simulink model "softMBD_old"  (R2025b)
settings: Solver=FixedStepAuto  StartTime=0.0  StopTime=10  FixedStep=0.005  RelTol=1e-3
values from neighbouring files (symbols this model uses):
  FPV_mass = 0.8    [Soft.m]
  g = 9.81    [Soft.m]
  ks = 0    [Soft.m]
  p_0 = 1013.25    [Soft.m]
  Q2Ts = forcetomotors()    [Soft.m]    (also in forcetomotors.m = inv(Ts2Q))
  takeOffDuration = 2    [Soft.m]
  Ts = 0.005    [Soft.m]
undefined symbols (not defined in the file or in its folder): DiscIntNeverNeededParam, kd_pq, kd_pr, kd_y, ki_pq, ki_pr, ki_t, ki_y, kp_pq, kp_pr, kp_y, pInitialization
libraries: simulink x35, discretizing x11, slpidlib x2, shared6dof x1, dynamicsLibrary x1, aerolibasang x1, aerolibnav x1
(part 18 of 20)

== system softMBD_old/FCS/filters/Subsystem1/roll_kalman/Kalman Filter/CalculatePL ==
  A : Inport
  C : Inport  Port=2
  Qbar : Inport  Port=3
  Rbar : Inport  Port=4
  Nbar : Inport  Port=5
  Enable : Inport  Port=6
  P[k-1] : Inport  Port=7
  CovarianceZ : Constant  Value=pInitialization.Z
  DataTypeConversionL : Subsystem  AncestorBlock=|  mask(Conversion Inherited){ConvertRealWorld=Real World Value, RndMeth=Floor, DoSatur=off}
      | simulink/Signal
      | Attributes/Data Type
      | Conversion
      | Inherited
      mask prompts: ConvertRealWorld "Simulink:masks:InputAndOutputToHaveEqual_MP"; RndMeth "Simulink:masks:IntegerRoundingMode_MP"; DoSatur "Simulink:masks:SaturateToMaxOrMinWhenOverflowsOccur_MP"
      mask help: Simulink:masks:ConversionInherited_MD
      mask init: same as softMBD_old/FCS/filters/Subsystem1/pitch_kalman/Kalman Filter1/DataTypeConversionP
      mask TypeOptions ConvertRealWorld: Simulink:masks:RealWorldValue | Simulink:masks:StoredInteger
      mask TypeOptions RndMeth: Simulink:masks:Ceiling | Simulink:masks:Convergent | Simulink:masks:Floor | Simulink:masks:Nearest | Simulink:masks:Round | Simulink:masks:Simplest | Simulink:masks:Zero
      mask Display:
      | port_label('Input',2,'u');
      | port_label('Output',1,'y');
      |     if(get_param(gcbh,'ConvertRealWorld') == "Stored Integer")
      |        disp('SI')
      |     else
      |        disp('Convert')
      |     end
  DataTypeConversionM : Subsystem  AncestorBlock=|  mask(Conversion Inherited){ConvertRealWorld=Real World Value, RndMeth=Floor, DoSatur=off}
      | simulink/Signal
      | Attributes/Data Type
      | Conversion
      | Inherited
      mask prompts: ConvertRealWorld "Simulink:masks:InputAndOutputToHaveEqual_MP"; RndMeth "Simulink:masks:IntegerRoundingMode_MP"; DoSatur "Simulink:masks:SaturateToMaxOrMinWhenOverflowsOccur_MP"
      mask help: Simulink:masks:ConversionInherited_MD
      mask init: same as softMBD_old/FCS/filters/Subsystem1/pitch_kalman/Kalman Filter1/DataTypeConversionP
      mask TypeOptions ConvertRealWorld: Simulink:masks:RealWorldValue | Simulink:masks:StoredInteger
      mask TypeOptions RndMeth: Simulink:masks:Ceiling | Simulink:masks:Convergent | Simulink:masks:Floor | Simulink:masks:Nearest | Simulink:masks:Round | Simulink:masks:Simplest | Simulink:masks:Zero
      mask Display:
      | port_label('Input',2,'u');
      | port_label('Output',1,'y');
      |     if(get_param(gcbh,'ConvertRealWorld') == "Stored Integer")
      |        disp('SI')
      |     else
      |        disp('Convert')
      |     end
  DataTypeConversionP : Subsystem  AncestorBlock=|  mask(Conversion Inherited){ConvertRealWorld=Real World Value, RndMeth=Floor, DoSatur=off}
      | simulink/Signal
      | Attributes/Data Type
      | Conversion
      | Inherited
      mask prompts: ConvertRealWorld "Simulink:masks:InputAndOutputToHaveEqual_MP"; RndMeth "Simulink:masks:IntegerRoundingMode_MP"; DoSatur "Simulink:masks:SaturateToMaxOrMinWhenOverflowsOccur_MP"
      mask help: Simulink:masks:ConversionInherited_MD
      mask init: same as softMBD_old/FCS/filters/Subsystem1/pitch_kalman/Kalman Filter1/DataTypeConversionP
      mask TypeOptions ConvertRealWorld: Simulink:masks:RealWorldValue | Simulink:masks:StoredInteger
      mask TypeOptions RndMeth: Simulink:masks:Ceiling | Simulink:masks:Convergent | Simulink:masks:Floor | Simulink:masks:Nearest | Simulink:masks:Round | Simulink:masks:Simplest | Simulink:masks:Zero
      mask Display:
      | port_label('Input',2,'u');
      | port_label('Output',1,'y');
      |     if(get_param(gcbh,'ConvertRealWorld') == "Stored Integer")
      |        disp('SI')
      |     else
      |        disp('Convert')
      |     end
  DataTypeConversionZ : Subsystem  AncestorBlock=|  mask(Conversion Inherited){ConvertRealWorld=Real World Value, RndMeth=Floor, DoSatur=off}
      | simulink/Signal
      | Attributes/Data Type
      | Conversion
      | Inherited
      mask prompts: ConvertRealWorld "Simulink:masks:InputAndOutputToHaveEqual_MP"; RndMeth "Simulink:masks:IntegerRoundingMode_MP"; DoSatur "Simulink:masks:SaturateToMaxOrMinWhenOverflowsOccur_MP"
      mask help: Simulink:masks:ConversionInherited_MD
      mask init: same as softMBD_old/FCS/filters/Subsystem1/pitch_kalman/Kalman Filter1/DataTypeConversionP
      mask TypeOptions ConvertRealWorld: Simulink:masks:RealWorldValue | Simulink:masks:StoredInteger
      mask TypeOptions RndMeth: Simulink:masks:Ceiling | Simulink:masks:Convergent | Simulink:masks:Floor | Simulink:masks:Nearest | Simulink:masks:Round | Simulink:masks:Simplest | Simulink:masks:Zero
      mask Display:
      | port_label('Input',2,'u');
      | port_label('Output',1,'y');
      |     if(get_param(gcbh,'ConvertRealWorld') == "Stored Integer")
      |        disp('SI')
      |     else
      |        disp('Convert')
      |     end
  Ground : Subsystem  AncestorBlock=ctrlSharedLib/Utilities/Ground  mask(ctrlSharedLibGround){OutDataTypeStr=single, Dimensions=1}
      mask prompts: OutDataTypeStr "Simulink:blkprm_prompts:UNIFIEDDATATYPE"; Dimensions "Simulink:blkprm_prompts:SigSpecDims"
      mask TypeOptions OutDataTypeStr: Signal Specification/OutDataTypeStr
      mask TypeOptions Dimensions: Signal Specification/Dimensions
      mask DialogControl OutDataTypeStr Prompt: Data type:
      mask DialogControl Dimensions Prompt: Dimensions (-1 for inherited):
  KalmanGainL : Constant  Value=pInitialization.L
  KalmanGainM : Constant  Value=pInitialization.M
  Terminator{,2,4..8} (7 alike) : Terminator
  M : Outport  VectorParamsAs1DForOutWhenUnconnected=off
  L : Outport  Port=2  VectorParamsAs1DForOutWhenUnconnected=off
  Z : Outport  Port=3  VectorParamsAs1DForOutWhenUnconnected=off
  P : Outport  Port=4  VectorParamsAs1DForOutWhenUnconnected=off
  wires:
  DataTypeConversionP/1(y) -> P/1
  CovarianceZ/1 -> DataTypeConversionZ/2(u)
  DataTypeConversionZ/1(y) -> Z/1
  Ground/1(Out) -> DataTypeConversionP/2(u)
  DataTypeConversionM/1(y) -> M/1
  KalmanGainM/1 -> DataTypeConversionM/2(u)
  P[k-1]/1 -> Terminator8/1
  Enable/1 -> Terminator7/1
  KalmanGainL/1 -> DataTypeConversionL/2(u)
  DataTypeConversionL/1(y) -> L/1
  Nbar/1 -> Terminator6/1
  Rbar/1 -> Terminator5/1
  Qbar/1 -> Terminator4/1
  C/1 -> Terminator2/1, DataTypeConversionL/1(DTS reference), DataTypeConversionM/1(DTS reference), DataTypeConversionZ/1(DTS reference), DataTypeConversionP/1(DTS reference)
  A/1 -> Terminator/1

== system softMBD_old/FCS/filters/Subsystem1/roll_kalman/Kalman Filter/CalculateYhat ==
  u : Inport  SampleTime=pInitialization.Ts
  C : Inport  Port=2  SampleTime=pInitialization.Ts
  D : Inport  Port=3  SampleTime=pInitialization.Ts
  xhat : Inport  Port=4  SampleTime=pInitialization.Ts
  Ground : Subsystem  AncestorBlock=ctrlSharedLib/Utilities/Ground  mask(ctrlSharedLibGround){OutDataTypeStr=single, Dimensions=1}
      mask prompts: OutDataTypeStr "Simulink:blkprm_prompts:UNIFIEDDATATYPE"; Dimensions "Simulink:blkprm_prompts:SigSpecDims"
      mask TypeOptions OutDataTypeStr: Signal Specification/OutDataTypeStr
      mask TypeOptions Dimensions: Signal Specification/Dimensions
      mask DialogControl OutDataTypeStr Prompt: Data type:
      mask DialogControl Dimensions Prompt: Dimensions (-1 for inherited):
  TerminatorC : Terminator
  TerminatorD : Terminator
  Terminatoru : Terminator
  Terminatorxhat : Terminator
  y[.] : Outport  VectorParamsAs1DForOutWhenUnconnected=off
  wires:
  Ground/1(Out) -> y[.]/1
  u/1 -> Terminatoru/1
  D/1 -> TerminatorD/1
  xhat/1 -> Terminatorxhat/1
  C/1 -> TerminatorC/1

== system softMBD_old/FCS/filters/Subsystem1/roll_kalman/Kalman Filter/CovarianceOutputConfigurator ==
  Z : Inport
  P : Inport  Port=2
  TerminatorP : Terminator
  TerminatorZ : Terminator
  decideOutput : Subsystem  mask(outputZorP){}
  Covariance : Outport  VectorParamsAs1DForOutWhenUnconnected=off
  wires:
  decideOutput/1(P) -> Covariance/1
  P/1 -> TerminatorP/1
  Z/1 -> TerminatorZ/1, decideOutput/1(Z)

== system softMBD_old/FCS/filters/Subsystem1/roll_kalman/Kalman Filter/DataTypeConversionA ==
  typeRef : Inport
  u : Inport  Port=2
  Data Type Duplicate : DataTypeDuplicate
  u_ : Outport  VectorParamsAs1DForOutWhenUnconnected=off
  wires:
  typeRef/1 -> Data Type Duplicate/1
  u/1 -> Data Type Duplicate/2, u_/1

== system softMBD_old/FCS/filters/Subsystem1/roll_kalman/Kalman Filter/DataTypeConversionB ==
  typeRef : Inport
  u : Inport  Port=2
  Data Type Duplicate : DataTypeDuplicate
  u_ : Outport  VectorParamsAs1DForOutWhenUnconnected=off
  wires:
  typeRef/1 -> Data Type Duplicate/1
  u/1 -> Data Type Duplicate/2, u_/1

== system softMBD_old/FCS/filters/Subsystem1/roll_kalman/Kalman Filter/DataTypeConversionC ==
  typeRef : Inport
  u : Inport  Port=2
  Data Type Duplicate : DataTypeDuplicate
  u_ : Outport  VectorParamsAs1DForOutWhenUnconnected=off
  wires:
  typeRef/1 -> Data Type Duplicate/1
  u/1 -> Data Type Duplicate/2, u_/1

== system softMBD_old/FCS/filters/Subsystem1/roll_kalman/Kalman Filter/DataTypeConversionD ==
  typeRef : Inport
  u : Inport  Port=2
  Data Type Duplicate : DataTypeDuplicate
  u_ : Outport  VectorParamsAs1DForOutWhenUnconnected=off
  wires:
  typeRef/1 -> Data Type Duplicate/1
  u/1 -> Data Type Duplicate/2, u_/1

== system softMBD_old/FCS/filters/Subsystem1/roll_kalman/Kalman Filter/DataTypeConversionEnable ==
  u : Inport
  u_ : Outport  VectorParamsAs1DForOutWhenUnconnected=off
  wires:
  u/1 -> u_/1

== system softMBD_old/FCS/filters/Subsystem1/roll_kalman/Kalman Filter/DataTypeConversionG ==
  typeRef : Inport
  u : Inport  Port=2
  Data Type Duplicate : DataTypeDuplicate
  u_ : Outport  VectorParamsAs1DForOutWhenUnconnected=off
  wires:
  typeRef/1 -> Data Type Duplicate/1
  u/1 -> Data Type Duplicate/2, u_/1

== system softMBD_old/FCS/filters/Subsystem1/roll_kalman/Kalman Filter/DataTypeConversionH ==
  typeRef : Inport
  u : Inport  Port=2
  Data Type Duplicate : DataTypeDuplicate
  u_ : Outport  VectorParamsAs1DForOutWhenUnconnected=off
  wires:
  typeRef/1 -> Data Type Duplicate/1
  u/1 -> Data Type Duplicate/2, u_/1

== system softMBD_old/FCS/filters/Subsystem1/roll_kalman/Kalman Filter/DataTypeConversionN ==
  typeRef : Inport
  u : Inport  Port=2
  Data Type Duplicate : DataTypeDuplicate
  u_ : Outport  VectorParamsAs1DForOutWhenUnconnected=off
  wires:
  typeRef/1 -> Data Type Duplicate/1
  u/1 -> Data Type Duplicate/2, u_/1

== system softMBD_old/FCS/filters/Subsystem1/roll_kalman/Kalman Filter/DataTypeConversionP ==
  DTS reference : Inport
  u : Inport  Port=2
  Conversion : DataTypeConversion  SaturateOnIntegerOverflow=off  RndMeth=Floor  LockScale=on
  Data Type Duplicate : DataTypeDuplicate  DisableCoverage=on
  y : Outport
  wires:
  Conversion/1 -> Data Type Duplicate/2, y/1
  DTS reference/1 -> Data Type Duplicate/1
  u/1 -> Conversion/1

== system softMBD_old/FCS/filters/Subsystem1/roll_kalman/Kalman Filter/DataTypeConversionP0 ==
  typeRef : Inport
  u : Inport  Port=2
  Data Type Duplicate : DataTypeDuplicate
  u_ : Outport  VectorParamsAs1DForOutWhenUnconnected=off
  wires:
  typeRef/1 -> Data Type Duplicate/1
  u/1 -> Data Type Duplicate/2, u_/1

== system softMBD_old/FCS/filters/Subsystem1/roll_kalman/Kalman Filter/DataTypeConversionQ ==
  typeRef : Inport
  u : Inport  Port=2
  Data Type Duplicate : DataTypeDuplicate
  u_ : Outport  VectorParamsAs1DForOutWhenUnconnected=off
  wires:
  typeRef/1 -> Data Type Duplicate/1
  u/1 -> Data Type Duplicate/2, u_/1

== system softMBD_old/FCS/filters/Subsystem1/roll_kalman/Kalman Filter/DataTypeConversionR ==
  typeRef : Inport
  u : Inport  Port=2
  Data Type Duplicate : DataTypeDuplicate
  u_ : Outport  VectorParamsAs1DForOutWhenUnconnected=off
  wires:
  typeRef/1 -> Data Type Duplicate/1
  u/1 -> Data Type Duplicate/2, u_/1

== system softMBD_old/FCS/filters/Subsystem1/roll_kalman/Kalman Filter/DataTypeConversionReset ==
  u : Inport
  u_ : Outport  VectorParamsAs1DForOutWhenUnconnected=off
  wires:
  u/1 -> u_/1

== system softMBD_old/FCS/filters/Subsystem1/roll_kalman/Kalman Filter/DataTypeConversionX ==
  DTS reference : Inport
  u : Inport  Port=2
  Conversion : DataTypeConversion  SaturateOnIntegerOverflow=off  RndMeth=Floor  LockScale=on
  Data Type Duplicate : DataTypeDuplicate  DisableCoverage=on
  y : Outport
  wires:
  Conversion/1 -> Data Type Duplicate/2, y/1
  DTS reference/1 -> Data Type Duplicate/1
  u/1 -> Conversion/1

== system softMBD_old/FCS/filters/Subsystem1/roll_kalman/Kalman Filter/DataTypeConversionX0 ==
  typeRef : Inport
  u : Inport  Port=2
  Data Type Duplicate : DataTypeDuplicate
  u_ : Outport  VectorParamsAs1DForOutWhenUnconnected=off
  wires:
  typeRef/1 -> Data Type Duplicate/1
  u/1 -> Data Type Duplicate/2, u_/1

== system softMBD_old/FCS/filters/Subsystem1/roll_kalman/Kalman Filter/DataTypeConversionu ==
  In1 : Inport
  u : Inport  Port=2
  Terminator : Terminator
  u_ : Outport  VectorParamsAs1DForOutWhenUnconnected=off
  wires:
  In1/1 -> Terminator/1
  u/1 -> u_/1

== system softMBD_old/FCS/filters/Subsystem1/roll_kalman/Kalman Filter/MemoryP ==
  T : Inport
  P : Inport  Port=2
  Terminator : Terminator
  P_ : Outport  VectorParamsAs1DForOutWhenUnconnected=off
  wires:
  T/1 -> Terminator/1
  P/1 -> P_/1

== system softMBD_old/FCS/filters/Subsystem1/roll_kalman/Kalman Filter/Observer ==
  note: A*xhat+B*u+L*(yMeas-yHat)
      | or
      | A*xhat+B*u
  u[k] : Inport  SampleTime=pInitialization.Ts
  y[k] : Inport  Port=2  SampleTime=pInitialization.Ts
  A[k] : Inport  Port=3  SampleTime=pInitialization.Ts
  B[k] : Inport  Port=4  SampleTime=pInitialization.Ts
  C[k] : Inport  Port=5  SampleTime=pInitialization.Ts
  D[k] : Inport  Port=6  SampleTime=pInitialization.Ts
  L[k] : Inport  Port=7  SampleTime=pInitialization.Ts
  Enable : Inport  Port=8  SampleTime=pInitialization.Ts
  xhat[k|k-1] : Inport  Port=9  SampleTime=pInitialization.Ts
  A[k]*xhat[k|k-1] : Product  Multiplication=Matrix(*)
  Add : Sum  Inputs=+++
  B[k]*u[k] : Product  Multiplication=Matrix(*)
  MeasurementUpdate : Subsystem  TreatAsAtomicUnit=on
  Reshape : Reshape
  x[k+1|k] : Outport  SampleTime=pInitialization.Ts  VectorParamsAs1DForOutWhenUnconnected=off
  wires:
  D[k]/1 -> MeasurementUpdate/5(D[k])
  Reshape/1 -> x[k+1|k]/1
  y[k]/1 -> MeasurementUpdate/2(y[k])
  C[k]/1 -> MeasurementUpdate/3(C[k])
  MeasurementUpdate/1(L*(y[k]-yhat[k|k-1])) -> Add/3
  A[k]/1 -> A[k]*xhat[k|k-1]/1
  xhat[k|k-1]/1 -> A[k]*xhat[k|k-1]/2, MeasurementUpdate/4(xhat[k|k-1])
  B[k]/1 -> B[k]*u[k]/1
  L[k]/1 -> MeasurementUpdate/1(L[k])
  A[k]*xhat[k|k-1]/1 -> Add/2
  u[k]/1 -> B[k]*u[k]/2, MeasurementUpdate/6(u[k])
  Add/1 -> Reshape/1
  B[k]*u[k]/1 -> Add/1
  Enable/1 -> MeasurementUpdate/Enable

== system softMBD_old/FCS/filters/Subsystem1/roll_kalman/Kalman Filter/ReducedQRN ==
  G : Inport  SampleTime=pInitialization.Ts
  H : Inport  Port=2  SampleTime=pInitialization.Ts
  Q : Inport  Port=3  SampleTime=pInitialization.Ts
  R : Inport  Port=4  SampleTime=pInitialization.Ts
  N : Inport  Port=5  SampleTime=pInitialization.Ts
  Ground : Subsystem  AncestorBlock=ctrlSharedLib/Utilities/Ground  mask(ctrlSharedLibGround){OutDataTypeStr=single, Dimensions=1}
      mask prompts: OutDataTypeStr "Simulink:blkprm_prompts:UNIFIEDDATATYPE"; Dimensions "Simulink:blkprm_prompts:SigSpecDims"
      mask TypeOptions OutDataTypeStr: Signal Specification/OutDataTypeStr
      mask TypeOptions Dimensions: Signal Specification/Dimensions
      mask DialogControl OutDataTypeStr Prompt: Data type:
      mask DialogControl Dimensions Prompt: Dimensions (-1 for inherited):
  Terminator{,1..4} (5 alike) : Terminator
  Qbar : Outport  SampleTime=pInitialization.Ts  VectorParamsAs1DForOutWhenUnconnected=off
  Rbar : Outport  Port=2  SampleTime=pInitialization.Ts  VectorParamsAs1DForOutWhenUnconnected=off
  Nbar : Outport  Port=3  SampleTime=pInitialization.Ts  VectorParamsAs1DForOutWhenUnconnected=off
  wires:
  Ground/1(Out) -> Rbar/1, Nbar/1, Qbar/1
  N/1 -> Terminator4/1
  R/1 -> Terminator3/1
  Q/1 -> Terminator2/1
  H/1 -> Terminator1/1
  G/1 -> Terminator/1

== system softMBD_old/FCS/filters/Subsystem1/roll_kalman/Kalman Filter/Reset ==
  note: Specification is to avoid underspecified data type warnings in the code generation process
  Ground : Ground
  Signal Specification : SignalSpecification  OutDataTypeStr=boolean  Dimensions=1
  Out : Outport  VectorParamsAs1DForOutWhenUnconnected=off
  wires:
  Signal Specification/1 -> Out/1
  Ground/1 -> Signal Specification/1

== system softMBD_old/FCS/filters/Subsystem1/roll_kalman/Kalman Filter/Reshapeyhat ==
  u : Inport
  u_ : Outport  VectorParamsAs1DForOutWhenUnconnected=off
  wires:
  u/1 -> u_/1

== system softMBD_old/FCS/filters/Subsystem1/roll_kalman/Kalman Filter/ScalarExpansionP0 ==
  u : Inport
  u_ : Outport  VectorParamsAs1DForOutWhenUnconnected=off
  wires:
  u/1 -> u_/1

== system softMBD_old/FCS/filters/Subsystem1/roll_kalman/Kalman Filter/ScalarExpansionQ ==
  u : Inport
  u_ : Outport  VectorParamsAs1DForOutWhenUnconnected=off
  wires:
  u/1 -> u_/1

== system softMBD_old/FCS/filters/Subsystem1/roll_kalman/Kalman Filter/ScalarExpansionR ==
  u : Inport
  u_ : Outport  VectorParamsAs1DForOutWhenUnconnected=off
  wires:
  u/1 -> u_/1

== system softMBD_old/FCS/filters/Subsystem1/roll_kalman/Kalman Filter/UseCurrentEstimator ==
  note: System model has D=0
      | Break connection, avoid fictitious algebraic loop
  Enable[k] : Inport  SampleTime=pInitialization.Ts
  M[k] : Inport  Port=2  SampleTime=pInitialization.Ts
  u (unused) : Inport  Port=3  SampleTime=pInitialization.Ts
  y[k] : Inport  Port=4  SampleTime=pInitialization.Ts
  C[k] : Inport  Port=5  SampleTime=pInitialization.Ts
  D (unused) : Inport  Port=6  SampleTime=pInitialization.Ts
  xhat[k|k-1] : Inport  Port=7  SampleTime=pInitialization.Ts
  Add : Sum
  Enabled Subsystem : Subsystem  TreatAsAtomicUnit=on
  Terminator : Terminator
  Terminator1 : Terminator
  xhat[k|k] : Outport  SampleTime=pInitialization.Ts  VectorParamsAs1DForOutWhenUnconnected=off
  wires:
  Add/1 -> xhat[k|k]/1
  u (unused)/1 -> Terminator1/1
  D (unused)/1 -> Terminator/1
  M[k]/1 -> Enabled Subsystem/1(M[k])
  C[k]/1 -> Enabled Subsystem/2(C[k])
  y[k]/1 -> Enabled Subsystem/3(y[k])
  xhat[k|k-1]/1 -> Add/2, Enabled Subsystem/4(xhat[k|k-1])
  Enabled Subsystem/1(deltax) -> Add/1
  Enable[k]/1 -> Enabled Subsystem/Enable

== system softMBD_old/FCS/filters/Subsystem1/roll_kalman/Kalman Filter/checkA ==
  In1 : Inport
  u : Inport  Port=2
  Terminator : Terminator
  u_ : Outport  VectorParamsAs1DForOutWhenUnconnected=off
  wires:
  In1/1 -> Terminator/1
  u/1 -> u_/1

== system softMBD_old/FCS/filters/Subsystem1/roll_kalman/Kalman Filter/checkB ==
  In1 : Inport
  u : Inport  Port=2
  Terminator : Terminator
  u_ : Outport  VectorParamsAs1DForOutWhenUnconnected=off
  wires:
  In1/1 -> Terminator/1
  u/1 -> u_/1

== system softMBD_old/FCS/filters/Subsystem1/roll_kalman/Kalman Filter/checkC ==
  In1 : Inport
  u : Inport  Port=2
  Terminator : Terminator
  u_ : Outport  VectorParamsAs1DForOutWhenUnconnected=off
  wires:
  In1/1 -> Terminator/1
  u/1 -> u_/1

== system softMBD_old/FCS/filters/Subsystem1/roll_kalman/Kalman Filter/checkD ==
  In1 : Inport
  u : Inport  Port=2
  Terminator : Terminator
  u_ : Outport  VectorParamsAs1DForOutWhenUnconnected=off
  wires:
  In1/1 -> Terminator/1
  u/1 -> u_/1

== system softMBD_old/FCS/filters/Subsystem1/roll_kalman/Kalman Filter/checkEnable ==
  In1 : Inport
  u : Inport  Port=2
  Terminator : Terminator
  u_ : Outport  VectorParamsAs1DForOutWhenUnconnected=off
  wires:
  In1/1 -> Terminator/1
  u/1 -> u_/1

== system softMBD_old/FCS/filters/Subsystem1/roll_kalman/Kalman Filter/checkG ==
  In1 : Inport
  u : Inport  Port=2
  Terminator : Terminator
  u_ : Outport  VectorParamsAs1DForOutWhenUnconnected=off
  wires:
  In1/1 -> Terminator/1
  u/1 -> u_/1

== system softMBD_old/FCS/filters/Subsystem1/roll_kalman/Kalman Filter/checkH ==
  In1 : Inport
  u : Inport  Port=2
  Terminator : Terminator
  u_ : Outport  VectorParamsAs1DForOutWhenUnconnected=off
  wires:
  In1/1 -> Terminator/1
  u/1 -> u_/1

== system softMBD_old/FCS/filters/Subsystem1/roll_kalman/Kalman Filter/checkN ==
  In1 : Inport
  u : Inport  Port=2
  Terminator : Terminator
  u_ : Outport  VectorParamsAs1DForOutWhenUnconnected=off
  wires:
  In1/1 -> Terminator/1
  u/1 -> u_/1

== system softMBD_old/FCS/filters/Subsystem1/roll_kalman/Kalman Filter/checkP0 ==
  In1 : Inport
  u : Inport  Port=2
  Terminator : Terminator
  u_ : Outport  VectorParamsAs1DForOutWhenUnconnected=off
  wires:
  In1/1 -> Terminator/1
  u/1 -> u_/1

== system softMBD_old/FCS/filters/Subsystem1/roll_kalman/Kalman Filter/checkQ ==
  In1 : Inport
  u : Inport  Port=2
  Terminator : Terminator
  u_ : Outport  VectorParamsAs1DForOutWhenUnconnected=off
  wires:
  In1/1 -> Terminator/1
  u/1 -> u_/1

== system softMBD_old/FCS/filters/Subsystem1/roll_kalman/Kalman Filter/checkR ==
  In1 : Inport
  u : Inport  Port=2
  Terminator : Terminator
  u_ : Outport  VectorParamsAs1DForOutWhenUnconnected=off
  wires:
  In1/1 -> Terminator/1
  u/1 -> u_/1

== system softMBD_old/FCS/filters/Subsystem1/roll_kalman/Kalman Filter/checkReset ==
  In1 : Inport
  u : Inport  Port=2
  Terminator : Terminator
  u_ : Outport  VectorParamsAs1DForOutWhenUnconnected=off
  wires:
  In1/1 -> Terminator/1
  u/1 -> u_/1

== system softMBD_old/FCS/filters/Subsystem1/roll_kalman/Kalman Filter/checkX0 ==
  In1 : Inport
  u : Inport  Port=2
  Terminator : Terminator
  u_ : Outport  VectorParamsAs1DForOutWhenUnconnected=off
  wires:
  In1/1 -> Terminator/1
  u/1 -> u_/1

== system softMBD_old/FCS/filters/Subsystem1/roll_kalman/Kalman Filter/checku ==
  Ref : Inport
  u : Inport  Port=2
  CheckSignalProperties : S-Function  FunctionName=ctrlKalmanFilterCheckSignals  Parameters=parentBlockPath,portName,isContinuousTime,pInitialization.Ts,Ns,Nu,Nw,Ny  SFunctionDeploymentMode=off  EnableBusSupport=off
  Data Type Conversion3 : DataTypeConversion  OutDataTypeStr=single  SaturateOnIntegerOverflow=off  RndMeth=Floor
  y : Outport  VectorParamsAs1DForOutWhenUnconnected=off
  wires:
  u/1 -> CheckSignalProperties/2, y/1
  Ref/1 -> Data Type Conversion3/1
  Data Type Conversion3/1 -> CheckSignalProperties/1

== system softMBD_old/FCS/filters/Subsystem1/roll_kalman/Kalman Filter/checky ==
  Ref : Inport
  u : Inport  Port=2
  CheckSignalProperties : S-Function  FunctionName=ctrlKalmanFilterCheckSignals  Parameters=parentBlockPath,portName,isContinuousTime,pInitialization.Ts,Ns,Nu,Nw,Ny  SFunctionDeploymentMode=off  EnableBusSupport=off
  y : Outport  VectorParamsAs1DForOutWhenUnconnected=off
  wires:
  u/1 -> CheckSignalProperties/2, y/1
  Ref/1 -> CheckSignalProperties/1

== system softMBD_old/FCS/Controller/position_controller/PID Controller/Anti-windup/Cont. Clamping Ideal/Dead Zone ==
  preSat : Inport
  Upper Limit : Inport  Port=2  SampleTime=SampleTime
  Lower Limit : Inport  Port=3  SampleTime=SampleTime
  Disabled : Subsystem  VariantControl=Disabled
  Enabled : Subsystem  VariantControl=Enabled
  External : Subsystem  VariantControl=External
  DZ out : Outport

== system softMBD_old/FCS/Controller/position_controller/PID Controller/Anti-windup/Cont. Clamping Parallel/Dead Zone ==
  preSat : Inport
  Upper Limit : Inport  Port=2  SampleTime=SampleTime
  Lower Limit : Inport  Port=3  SampleTime=SampleTime
  Disabled : Subsystem  VariantControl=Disabled
  Enabled : Subsystem  VariantControl=Enabled
  External : Subsystem  VariantControl=External
  DZ out : Outport

== system softMBD_old/FCS/Controller/position_controller/PID Controller/Anti-windup/Disc. Clamping Ideal/Dead Zone ==
  preSat : Inport
  Upper Limit : Inport  Port=2  SampleTime=SampleTime
  Lower Limit : Inport  Port=3  SampleTime=SampleTime
  Disabled : Subsystem  VariantControl=Disabled
  Enabled : Subsystem  VariantControl=Enabled
  External : Subsystem  VariantControl=External
  DZ out : Outport

== system softMBD_old/FCS/Controller/position_controller/PID Controller/Anti-windup/Disc. Clamping Parallel/Dead Zone ==
  preSat : Inport
  Upper Limit : Inport  Port=2  SampleTime=SampleTime
  Lower Limit : Inport  Port=3  SampleTime=SampleTime
  Disabled : Subsystem  VariantControl=Disabled
  Enabled : Subsystem  VariantControl=Enabled
  External : Subsystem  VariantControl=External
  DZ out : Outport

== system softMBD_old/FCS/Controller/position_controller/PID Controller/Filter/Differentiator/Tsamp ==
  U : Inport  SampleTime=SampleTime
  Ts : Inport  Port=2  SampleTime=SampleTime
  External Ts : Subsystem  VariantControl=ExternalTs
  Internal Ts : Subsystem  VariantControl=InternalTs
  Out1 : Outport  SampleTime=SampleTime

== system softMBD_old/FCS/Controller/position_controller/PID Controller/Filter/Disc. Backward Euler Filter/Tsamp ==
  N : Inport  SampleTime=SampleTime
  Ts : Inport  Port=2  SampleTime=SampleTime
  External Ts : Subsystem  VariantControl=ExternalTs
  Internal Ts : Subsystem  VariantControl=InternalTs
  Out1 : Outport  SampleTime=SampleTime

== system softMBD_old/FCS/Controller/position_controller/PID Controller/Filter/Disc. Backward Euler Filter Only/Tsamp ==
  N : Inport  SampleTime=SampleTime
  Ts : Inport  Port=2  SampleTime=SampleTime
  External Ts : Subsystem  VariantControl=ExternalTs
  Internal Ts : Subsystem  VariantControl=InternalTs
  Out1 : Outport  SampleTime=SampleTime

== system softMBD_old/FCS/Controller/position_controller/PID Controller/Filter/Disc. Trapezoidal Filter/Tsamp ==
  N : Inport  SampleTime=SampleTime
  Ts : Inport  Port=2  SampleTime=SampleTime
  External Ts : Subsystem  VariantControl=ExternalTs
  Internal Ts : Subsystem  VariantControl=InternalTs
  Out1 : Outport  SampleTime=SampleTime

== system softMBD_old/FCS/Controller/position_controller/PID Controller/Filter/Disc. Trapezoidal Filter Only/Tsamp ==
  N : Inport  SampleTime=SampleTime
  Ts : Inport  Port=2  SampleTime=SampleTime
  External Ts : Subsystem  VariantControl=ExternalTs
  Internal Ts : Subsystem  VariantControl=InternalTs
  Out1 : Outport  SampleTime=SampleTime

== system softMBD_old/FCS/Controller/position_controller/PID Controller1/Anti-windup/Cont. Clamping Ideal/Dead Zone ==
  preSat : Inport
  Upper Limit : Inport  Port=2  SampleTime=SampleTime
  Lower Limit : Inport  Port=3  SampleTime=SampleTime
  Disabled : Subsystem  VariantControl=Disabled
  Enabled : Subsystem  VariantControl=Enabled
  External : Subsystem  VariantControl=External
  DZ out : Outport

== system softMBD_old/FCS/Controller/position_controller/PID Controller1/Anti-windup/Cont. Clamping Parallel/Dead Zone ==
  preSat : Inport
  Upper Limit : Inport  Port=2  SampleTime=SampleTime
  Lower Limit : Inport  Port=3  SampleTime=SampleTime
  Disabled : Subsystem  VariantControl=Disabled
  Enabled : Subsystem  VariantControl=Enabled
  External : Subsystem  VariantControl=External
  DZ out : Outport

== system softMBD_old/FCS/Controller/position_controller/PID Controller1/Anti-windup/Disc. Clamping Ideal/Dead Zone ==
  preSat : Inport
  Upper Limit : Inport  Port=2  SampleTime=SampleTime
  Lower Limit : Inport  Port=3  SampleTime=SampleTime
  Disabled : Subsystem  VariantControl=Disabled
  Enabled : Subsystem  VariantControl=Enabled
  External : Subsystem  VariantControl=External
  DZ out : Outport

== system softMBD_old/FCS/Controller/position_controller/PID Controller1/Anti-windup/Disc. Clamping Parallel/Dead Zone ==
  preSat : Inport
  Upper Limit : Inport  Port=2  SampleTime=SampleTime
  Lower Limit : Inport  Port=3  SampleTime=SampleTime
  Disabled : Subsystem  VariantControl=Disabled
  Enabled : Subsystem  VariantControl=Enabled
  External : Subsystem  VariantControl=External
  DZ out : Outport

== system softMBD_old/FCS/Controller/position_controller/PID Controller1/Filter/Differentiator/Tsamp ==
  U : Inport  SampleTime=SampleTime
  Ts : Inport  Port=2  SampleTime=SampleTime
  External Ts : Subsystem  VariantControl=ExternalTs
  Internal Ts : Subsystem  VariantControl=InternalTs
  Out1 : Outport  SampleTime=SampleTime

== system softMBD_old/FCS/Controller/position_controller/PID Controller1/Filter/Disc. Backward Euler Filter/Tsamp ==
  N : Inport  SampleTime=SampleTime
  Ts : Inport  Port=2  SampleTime=SampleTime
  External Ts : Subsystem  VariantControl=ExternalTs
  Internal Ts : Subsystem  VariantControl=InternalTs
  Out1 : Outport  SampleTime=SampleTime

== system softMBD_old/FCS/Controller/position_controller/PID Controller1/Filter/Disc. Backward Euler Filter Only/Tsamp ==
  N : Inport  SampleTime=SampleTime
  Ts : Inport  Port=2  SampleTime=SampleTime
  External Ts : Subsystem  VariantControl=ExternalTs
  Internal Ts : Subsystem  VariantControl=InternalTs
  Out1 : Outport  SampleTime=SampleTime

== system softMBD_old/FCS/Controller/position_controller/PID Controller1/Filter/Disc. Trapezoidal Filter/Tsamp ==
  N : Inport  SampleTime=SampleTime
  Ts : Inport  Port=2  SampleTime=SampleTime
  External Ts : Subsystem  VariantControl=ExternalTs
  Internal Ts : Subsystem  VariantControl=InternalTs
  Out1 : Outport  SampleTime=SampleTime

== system softMBD_old/FCS/Controller/position_controller/PID Controller1/Filter/Disc. Trapezoidal Filter Only/Tsamp ==
  N : Inport  SampleTime=SampleTime
  Ts : Inport  Port=2  SampleTime=SampleTime
  External Ts : Subsystem  VariantControl=ExternalTs
  Internal Ts : Subsystem  VariantControl=InternalTs
  Out1 : Outport  SampleTime=SampleTime

== system softMBD_old/FCS/Controller/position_controller/PID Controller2/Anti-windup/Cont. Clamping Ideal/Dead Zone ==
  preSat : Inport
  Upper Limit : Inport  Port=2  SampleTime=SampleTime
  Lower Limit : Inport  Port=3  SampleTime=SampleTime
  Disabled : Subsystem  VariantControl=Disabled
  Enabled : Subsystem  VariantControl=Enabled
  External : Subsystem  VariantControl=External
  DZ out : Outport

== system softMBD_old/FCS/Controller/position_controller/PID Controller2/Anti-windup/Cont. Clamping Parallel/Dead Zone ==
  preSat : Inport
  Upper Limit : Inport  Port=2  SampleTime=SampleTime
  Lower Limit : Inport  Port=3  SampleTime=SampleTime
  Disabled : Subsystem  VariantControl=Disabled
  Enabled : Subsystem  VariantControl=Enabled
  External : Subsystem  VariantControl=External
  DZ out : Outport

== system softMBD_old/FCS/Controller/position_controller/PID Controller2/Anti-windup/Disc. Clamping Ideal/Dead Zone ==
  preSat : Inport
  Upper Limit : Inport  Port=2  SampleTime=SampleTime
  Lower Limit : Inport  Port=3  SampleTime=SampleTime
  Disabled : Subsystem  VariantControl=Disabled
  Enabled : Subsystem  VariantControl=Enabled
  External : Subsystem  VariantControl=External
  DZ out : Outport

== system softMBD_old/FCS/Controller/position_controller/PID Controller2/Anti-windup/Disc. Clamping Parallel/Dead Zone ==
  preSat : Inport
  Upper Limit : Inport  Port=2  SampleTime=SampleTime
  Lower Limit : Inport  Port=3  SampleTime=SampleTime
  Disabled : Subsystem  VariantControl=Disabled
  Enabled : Subsystem  VariantControl=Enabled
  External : Subsystem  VariantControl=External
  DZ out : Outport

== system softMBD_old/FCS/Controller/position_controller/PID Controller2/Filter/Differentiator/Tsamp ==
  U : Inport  SampleTime=SampleTime
  Ts : Inport  Port=2  SampleTime=SampleTime
  External Ts : Subsystem  VariantControl=ExternalTs
  Internal Ts : Subsystem  VariantControl=InternalTs
  Out1 : Outport  SampleTime=SampleTime

== system softMBD_old/FCS/Controller/position_controller/PID Controller2/Filter/Disc. Backward Euler Filter/Tsamp ==
  N : Inport  SampleTime=SampleTime
  Ts : Inport  Port=2  SampleTime=SampleTime
  External Ts : Subsystem  VariantControl=ExternalTs
  Internal Ts : Subsystem  VariantControl=InternalTs
  Out1 : Outport  SampleTime=SampleTime

== system softMBD_old/FCS/Controller/position_controller/PID Controller2/Filter/Disc. Backward Euler Filter Only/Tsamp ==
  N : Inport  SampleTime=SampleTime
  Ts : Inport  Port=2  SampleTime=SampleTime
  External Ts : Subsystem  VariantControl=ExternalTs
  Internal Ts : Subsystem  VariantControl=InternalTs
  Out1 : Outport  SampleTime=SampleTime

== system softMBD_old/FCS/Controller/position_controller/PID Controller2/Filter/Disc. Trapezoidal Filter/Tsamp ==
  N : Inport  SampleTime=SampleTime
  Ts : Inport  Port=2  SampleTime=SampleTime
  External Ts : Subsystem  VariantControl=ExternalTs
  Internal Ts : Subsystem  VariantControl=InternalTs
  Out1 : Outport  SampleTime=SampleTime

== system softMBD_old/FCS/Controller/position_controller/PID Controller2/Filter/Disc. Trapezoidal Filter Only/Tsamp ==
  N : Inport  SampleTime=SampleTime
  Ts : Inport  Port=2  SampleTime=SampleTime
  External Ts : Subsystem  VariantControl=ExternalTs
  Internal Ts : Subsystem  VariantControl=InternalTs
  Out1 : Outport  SampleTime=SampleTime

== system softMBD_old/FCS/Controller/position_controller/PID Controller3/Anti-windup/Cont. Clamping Ideal/Dead Zone ==
  preSat : Inport
  Upper Limit : Inport  Port=2  SampleTime=SampleTime
  Lower Limit : Inport  Port=3  SampleTime=SampleTime
  Disabled : Subsystem  VariantControl=Disabled
  Enabled : Subsystem  VariantControl=Enabled
  External : Subsystem  VariantControl=External
  DZ out : Outport

== system softMBD_old/FCS/Controller/position_controller/PID Controller3/Anti-windup/Cont. Clamping Parallel/Dead Zone ==
  preSat : Inport
  Upper Limit : Inport  Port=2  SampleTime=SampleTime
  Lower Limit : Inport  Port=3  SampleTime=SampleTime
  Disabled : Subsystem  VariantControl=Disabled
  Enabled : Subsystem  VariantControl=Enabled
  External : Subsystem  VariantControl=External
  DZ out : Outport

== system softMBD_old/FCS/Controller/position_controller/PID Controller3/Anti-windup/Disc. Clamping Ideal/Dead Zone ==
  preSat : Inport
  Upper Limit : Inport  Port=2  SampleTime=SampleTime
  Lower Limit : Inport  Port=3  SampleTime=SampleTime
  Disabled : Subsystem  VariantControl=Disabled
  Enabled : Subsystem  VariantControl=Enabled
  External : Subsystem  VariantControl=External
  DZ out : Outport

== system softMBD_old/FCS/Controller/position_controller/PID Controller3/Anti-windup/Disc. Clamping Parallel/Dead Zone ==
  preSat : Inport
  Upper Limit : Inport  Port=2  SampleTime=SampleTime
  Lower Limit : Inport  Port=3  SampleTime=SampleTime
  Disabled : Subsystem  VariantControl=Disabled
  Enabled : Subsystem  VariantControl=Enabled
  External : Subsystem  VariantControl=External
  DZ out : Outport

== system softMBD_old/FCS/Controller/position_controller/PID Controller3/Filter/Differentiator/Tsamp ==
  U : Inport  SampleTime=SampleTime
  Ts : Inport  Port=2  SampleTime=SampleTime
  External Ts : Subsystem  VariantControl=ExternalTs
  Internal Ts : Subsystem  VariantControl=InternalTs
  Out1 : Outport  SampleTime=SampleTime

== system softMBD_old/FCS/Controller/position_controller/PID Controller3/Filter/Disc. Backward Euler Filter/Tsamp ==
  N : Inport  SampleTime=SampleTime
  Ts : Inport  Port=2  SampleTime=SampleTime
  External Ts : Subsystem  VariantControl=ExternalTs
  Internal Ts : Subsystem  VariantControl=InternalTs
  Out1 : Outport  SampleTime=SampleTime

== system softMBD_old/FCS/Controller/position_controller/PID Controller3/Filter/Disc. Backward Euler Filter Only/Tsamp ==
  N : Inport  SampleTime=SampleTime
  Ts : Inport  Port=2  SampleTime=SampleTime
  External Ts : Subsystem  VariantControl=ExternalTs
  Internal Ts : Subsystem  VariantControl=InternalTs
  Out1 : Outport  SampleTime=SampleTime

== system softMBD_old/FCS/Controller/position_controller/PID Controller3/Filter/Disc. Trapezoidal Filter/Tsamp ==
  N : Inport  SampleTime=SampleTime
  Ts : Inport  Port=2  SampleTime=SampleTime
  External Ts : Subsystem  VariantControl=ExternalTs
  Internal Ts : Subsystem  VariantControl=InternalTs
  Out1 : Outport  SampleTime=SampleTime

== system softMBD_old/FCS/Controller/position_controller/PID Controller3/Filter/Disc. Trapezoidal Filter Only/Tsamp ==
  N : Inport  SampleTime=SampleTime
  Ts : Inport  Port=2  SampleTime=SampleTime
  External Ts : Subsystem  VariantControl=ExternalTs
  Internal Ts : Subsystem  VariantControl=InternalTs
  Out1 : Outport  SampleTime=SampleTime

== system softMBD_old/FCS/Controller/roll_pitch_controller/PID Controller/Anti-windup/Cont. Clamping Ideal/Dead Zone ==
  preSat : Inport
  Upper Limit : Inport  Port=2  SampleTime=SampleTime
  Lower Limit : Inport  Port=3  SampleTime=SampleTime
  Disabled : Subsystem  VariantControl=Disabled
  Enabled : Subsystem  VariantControl=Enabled
  External : Subsystem  VariantControl=External
  DZ out : Outport

== system softMBD_old/FCS/Controller/roll_pitch_controller/PID Controller/Anti-windup/Cont. Clamping Parallel/Dead Zone ==
  preSat : Inport
  Upper Limit : Inport  Port=2  SampleTime=SampleTime
  Lower Limit : Inport  Port=3  SampleTime=SampleTime
  Disabled : Subsystem  VariantControl=Disabled
  Enabled : Subsystem  VariantControl=Enabled
  External : Subsystem  VariantControl=External
  DZ out : Outport

== system softMBD_old/FCS/Controller/roll_pitch_controller/PID Controller/Anti-windup/Disc. Clamping Ideal/Dead Zone ==
  preSat : Inport
  Upper Limit : Inport  Port=2  SampleTime=SampleTime
  Lower Limit : Inport  Port=3  SampleTime=SampleTime
  Disabled : Subsystem  VariantControl=Disabled
  Enabled : Subsystem  VariantControl=Enabled
  External : Subsystem  VariantControl=External
  DZ out : Outport

== system softMBD_old/FCS/Controller/roll_pitch_controller/PID Controller/Anti-windup/Disc. Clamping Parallel/Dead Zone ==
  preSat : Inport
  Upper Limit : Inport  Port=2  SampleTime=SampleTime
  Lower Limit : Inport  Port=3  SampleTime=SampleTime
  Disabled : Subsystem  VariantControl=Disabled
  Enabled : Subsystem  VariantControl=Enabled
  External : Subsystem  VariantControl=External
  DZ out : Outport

== system softMBD_old/FCS/Controller/roll_pitch_controller/PID Controller/Filter/Differentiator/Tsamp ==
  U : Inport  SampleTime=SampleTime
  Ts : Inport  Port=2  SampleTime=SampleTime
  External Ts : Subsystem  VariantControl=ExternalTs
  Internal Ts : Subsystem  VariantControl=InternalTs
  Out1 : Outport  SampleTime=SampleTime

== system softMBD_old/FCS/Controller/roll_pitch_controller/PID Controller/Filter/Disc. Backward Euler Filter/Tsamp ==
  N : Inport  SampleTime=SampleTime
  Ts : Inport  Port=2  SampleTime=SampleTime
  External Ts : Subsystem  VariantControl=ExternalTs
  Internal Ts : Subsystem  VariantControl=InternalTs
  Out1 : Outport  SampleTime=SampleTime

== system softMBD_old/FCS/Controller/roll_pitch_controller/PID Controller/Filter/Disc. Backward Euler Filter Only/Tsamp ==
  N : Inport  SampleTime=SampleTime
  Ts : Inport  Port=2  SampleTime=SampleTime
  External Ts : Subsystem  VariantControl=ExternalTs
  Internal Ts : Subsystem  VariantControl=InternalTs
  Out1 : Outport  SampleTime=SampleTime

== system softMBD_old/FCS/Controller/roll_pitch_controller/PID Controller/Filter/Disc. Trapezoidal Filter/Tsamp ==
  N : Inport  SampleTime=SampleTime
  Ts : Inport  Port=2  SampleTime=SampleTime
  External Ts : Subsystem  VariantControl=ExternalTs
  Internal Ts : Subsystem  VariantControl=InternalTs
  Out1 : Outport  SampleTime=SampleTime

== system softMBD_old/FCS/Controller/roll_pitch_controller/PID Controller/Filter/Disc. Trapezoidal Filter Only/Tsamp ==
  N : Inport  SampleTime=SampleTime
  Ts : Inport  Port=2  SampleTime=SampleTime
  External Ts : Subsystem  VariantControl=ExternalTs
  Internal Ts : Subsystem  VariantControl=InternalTs
  Out1 : Outport  SampleTime=SampleTime

== system softMBD_old/FCS/filters/Subsystem/x,y,z,dy,dy,dz/z,dz/Kalman Filter1/CalculatePL ==
  A : Inport
  C : Inport  Port=2
  Qbar : Inport  Port=3
  Rbar : Inport  Port=4
  Nbar : Inport  Port=5
  Enable : Inport  Port=6
  P[k-1] : Inport  Port=7
  CovarianceZ : Constant  Value=pInitialization.Z
  DataTypeConversionL : Subsystem  AncestorBlock=|  mask(Conversion Inherited){ConvertRealWorld=Real World Value, RndMeth=Floor, DoSatur=off}
      | simulink/Signal
      | Attributes/Data Type
      | Conversion
      | Inherited
      mask prompts: ConvertRealWorld "Simulink:masks:InputAndOutputToHaveEqual_MP"; RndMeth "Simulink:masks:IntegerRoundingMode_MP"; DoSatur "Simulink:masks:SaturateToMaxOrMinWhenOverflowsOccur_MP"
      mask help: Simulink:masks:ConversionInherited_MD
      mask init: same as softMBD_old/FCS/filters/Subsystem1/pitch_kalman/Kalman Filter1/DataTypeConversionP
      mask TypeOptions ConvertRealWorld: Simulink:masks:RealWorldValue | Simulink:masks:StoredInteger
      mask TypeOptions RndMeth: Simulink:masks:Ceiling | Simulink:masks:Convergent | Simulink:masks:Floor | Simulink:masks:Nearest | Simulink:masks:Round | Simulink:masks:Simplest | Simulink:masks:Zero
      mask Display:
      | port_label('Input',2,'u');
      | port_label('Output',1,'y');
      |     if(get_param(gcbh,'ConvertRealWorld') == "Stored Integer")
      |        disp('SI')
      |     else
      |        disp('Convert')
      |     end
  DataTypeConversionM : Subsystem  AncestorBlock=|  mask(Conversion Inherited){ConvertRealWorld=Real World Value, RndMeth=Floor, DoSatur=off}
      | simulink/Signal
      | Attributes/Data Type
      | Conversion
      | Inherited
      mask prompts: ConvertRealWorld "Simulink:masks:InputAndOutputToHaveEqual_MP"; RndMeth "Simulink:masks:IntegerRoundingMode_MP"; DoSatur "Simulink:masks:SaturateToMaxOrMinWhenOverflowsOccur_MP"
      mask help: Simulink:masks:ConversionInherited_MD
      mask init: same as softMBD_old/FCS/filters/Subsystem1/pitch_kalman/Kalman Filter1/DataTypeConversionP
      mask TypeOptions ConvertRealWorld: Simulink:masks:RealWorldValue | Simulink:masks:StoredInteger
      mask TypeOptions RndMeth: Simulink:masks:Ceiling | Simulink:masks:Convergent | Simulink:masks:Floor | Simulink:masks:Nearest | Simulink:masks:Round | Simulink:masks:Simplest | Simulink:masks:Zero
      mask Display:
      | port_label('Input',2,'u');
      | port_label('Output',1,'y');
      |     if(get_param(gcbh,'ConvertRealWorld') == "Stored Integer")
      |        disp('SI')
      |     else
      |        disp('Convert')
      |     end
  DataTypeConversionP : Subsystem  AncestorBlock=|  mask(Conversion Inherited){ConvertRealWorld=Real World Value, RndMeth=Floor, DoSatur=off}
      | simulink/Signal
      | Attributes/Data Type
      | Conversion
      | Inherited
      mask prompts: ConvertRealWorld "Simulink:masks:InputAndOutputToHaveEqual_MP"; RndMeth "Simulink:masks:IntegerRoundingMode_MP"; DoSatur "Simulink:masks:SaturateToMaxOrMinWhenOverflowsOccur_MP"
      mask help: Simulink:masks:ConversionInherited_MD
      mask init: same as softMBD_old/FCS/filters/Subsystem1/pitch_kalman/Kalman Filter1/DataTypeConversionP
      mask TypeOptions ConvertRealWorld: Simulink:masks:RealWorldValue | Simulink:masks:StoredInteger
      mask TypeOptions RndMeth: Simulink:masks:Ceiling | Simulink:masks:Convergent | Simulink:masks:Floor | Simulink:masks:Nearest | Simulink:masks:Round | Simulink:masks:Simplest | Simulink:masks:Zero
      mask Display:
      | port_label('Input',2,'u');
      | port_label('Output',1,'y');
      |     if(get_param(gcbh,'ConvertRealWorld') == "Stored Integer")
      |        disp('SI')
      |     else
      |        disp('Convert')
      |     end
  DataTypeConversionZ : Subsystem  AncestorBlock=|  mask(Conversion Inherited){ConvertRealWorld=Real World Value, RndMeth=Floor, DoSatur=off}
      | simulink/Signal
      | Attributes/Data Type
      | Conversion
      | Inherited
      mask prompts: ConvertRealWorld "Simulink:masks:InputAndOutputToHaveEqual_MP"; RndMeth "Simulink:masks:IntegerRoundingMode_MP"; DoSatur "Simulink:masks:SaturateToMaxOrMinWhenOverflowsOccur_MP"
      mask help: Simulink:masks:ConversionInherited_MD
      mask init: same as softMBD_old/FCS/filters/Subsystem1/pitch_kalman/Kalman Filter1/DataTypeConversionP
      mask TypeOptions ConvertRealWorld: Simulink:masks:RealWorldValue | Simulink:masks:StoredInteger
      mask TypeOptions RndMeth: Simulink:masks:Ceiling | Simulink:masks:Convergent | Simulink:masks:Floor | Simulink:masks:Nearest | Simulink:masks:Round | Simulink:masks:Simplest | Simulink:masks:Zero
      mask Display:
      | port_label('Input',2,'u');
      | port_label('Output',1,'y');
      |     if(get_param(gcbh,'ConvertRealWorld') == "Stored Integer")
      |        disp('SI')
      |     else
      |        disp('Convert')
      |     end
  Ground : Subsystem  AncestorBlock=ctrlSharedLib/Utilities/Ground  mask(ctrlSharedLibGround){OutDataTypeStr=single, Dimensions=1}
      mask prompts: OutDataTypeStr "Simulink:blkprm_prompts:UNIFIEDDATATYPE"; Dimensions "Simulink:blkprm_prompts:SigSpecDims"
      mask TypeOptions OutDataTypeStr: Signal Specification/OutDataTypeStr
      mask TypeOptions Dimensions: Signal Specification/Dimensions
      mask DialogControl OutDataTypeStr Prompt: Data type:
      mask DialogControl Dimensions Prompt: Dimensions (-1 for inherited):
  KalmanGainL : Constant  Value=pInitialization.L
  KalmanGainM : Constant  Value=pInitialization.M
  Terminator{,2,4..8} (7 alike) : Terminator
  M : Outport  VectorParamsAs1DForOutWhenUnconnected=off
  L : Outport  Port=2  VectorParamsAs1DForOutWhenUnconnected=off
  Z : Outport  Port=3  VectorParamsAs1DForOutWhenUnconnected=off
  P : Outport  Port=4  VectorParamsAs1DForOutWhenUnconnected=off
  wires:
  DataTypeConversionP/1(y) -> P/1
  CovarianceZ/1 -> DataTypeConversionZ/2(u)
  DataTypeConversionZ/1(y) -> Z/1
  Ground/1(Out) -> DataTypeConversionP/2(u)
  DataTypeConversionM/1(y) -> M/1
  KalmanGainM/1 -> DataTypeConversionM/2(u)
  P[k-1]/1 -> Terminator8/1
  Enable/1 -> Terminator7/1
  KalmanGainL/1 -> DataTypeConversionL/2(u)
  DataTypeConversionL/1(y) -> L/1
  Nbar/1 -> Terminator6/1
  Rbar/1 -> Terminator5/1
  Qbar/1 -> Terminator4/1
  C/1 -> Terminator2/1, DataTypeConversionL/1(DTS reference), DataTypeConversionM/1(DTS reference), DataTypeConversionZ/1(DTS reference), DataTypeConversionP/1(DTS reference)
  A/1 -> Terminator/1

== system softMBD_old/FCS/filters/Subsystem/x,y,z,dy,dy,dz/z,dz/Kalman Filter1/CalculateYhat ==
  u : Inport  SampleTime=pInitialization.Ts
  C : Inport  Port=2  SampleTime=pInitialization.Ts
  D : Inport  Port=3  SampleTime=pInitialization.Ts
  xhat : Inport  Port=4  SampleTime=pInitialization.Ts
  Ground : Subsystem  AncestorBlock=ctrlSharedLib/Utilities/Ground  mask(ctrlSharedLibGround){OutDataTypeStr=single, Dimensions=1}
      mask prompts: OutDataTypeStr "Simulink:blkprm_prompts:UNIFIEDDATATYPE"; Dimensions "Simulink:blkprm_prompts:SigSpecDims"
      mask TypeOptions OutDataTypeStr: Signal Specification/OutDataTypeStr
      mask TypeOptions Dimensions: Signal Specification/Dimensions
      mask DialogControl OutDataTypeStr Prompt: Data type:
      mask DialogControl Dimensions Prompt: Dimensions (-1 for inherited):
  TerminatorC : Terminator
  TerminatorD : Terminator
  Terminatoru : Terminator
  Terminatorxhat : Terminator
  y[.] : Outport  VectorParamsAs1DForOutWhenUnconnected=off
  wires:
  Ground/1(Out) -> y[.]/1
  u/1 -> Terminatoru/1
  D/1 -> TerminatorD/1
  xhat/1 -> Terminatorxhat/1
  C/1 -> TerminatorC/1

== system softMBD_old/FCS/filters/Subsystem/x,y,z,dy,dy,dz/z,dz/Kalman Filter1/CovarianceOutputConfigurator ==
  Z : Inport
  P : Inport  Port=2
  TerminatorP : Terminator
  TerminatorZ : Terminator
  decideOutput : Subsystem  mask(outputZorP){}
  Covariance : Outport  VectorParamsAs1DForOutWhenUnconnected=off
  wires:
  decideOutput/1(P) -> Covariance/1
  P/1 -> TerminatorP/1
  Z/1 -> TerminatorZ/1, decideOutput/1(Z)

== system softMBD_old/FCS/filters/Subsystem/x,y,z,dy,dy,dz/z,dz/Kalman Filter1/DataTypeConversionA ==
  typeRef : Inport
  u : Inport  Port=2
  Data Type Duplicate : DataTypeDuplicate
  u_ : Outport  VectorParamsAs1DForOutWhenUnconnected=off
  wires:
  typeRef/1 -> Data Type Duplicate/1
  u/1 -> Data Type Duplicate/2, u_/1

== system softMBD_old/FCS/filters/Subsystem/x,y,z,dy,dy,dz/z,dz/Kalman Filter1/DataTypeConversionB ==
  typeRef : Inport
  u : Inport  Port=2
  Data Type Duplicate : DataTypeDuplicate
  u_ : Outport  VectorParamsAs1DForOutWhenUnconnected=off
  wires:
  typeRef/1 -> Data Type Duplicate/1
  u/1 -> Data Type Duplicate/2, u_/1

== system softMBD_old/FCS/filters/Subsystem/x,y,z,dy,dy,dz/z,dz/Kalman Filter1/DataTypeConversionC ==
  typeRef : Inport
  u : Inport  Port=2
  Data Type Duplicate : DataTypeDuplicate
  u_ : Outport  VectorParamsAs1DForOutWhenUnconnected=off
  wires:
  typeRef/1 -> Data Type Duplicate/1
  u/1 -> Data Type Duplicate/2, u_/1

== system softMBD_old/FCS/filters/Subsystem/x,y,z,dy,dy,dz/z,dz/Kalman Filter1/DataTypeConversionD ==
  typeRef : Inport
  u : Inport  Port=2
  Data Type Duplicate : DataTypeDuplicate
  u_ : Outport  VectorParamsAs1DForOutWhenUnconnected=off
  wires:
  typeRef/1 -> Data Type Duplicate/1
  u/1 -> Data Type Duplicate/2, u_/1

== system softMBD_old/FCS/filters/Subsystem/x,y,z,dy,dy,dz/z,dz/Kalman Filter1/DataTypeConversionEnable ==
  u : Inport
  u_ : Outport  VectorParamsAs1DForOutWhenUnconnected=off
  wires:
  u/1 -> u_/1
